simulink model "Sine_Cases"  (R2023a)
settings: Solver=VariableStepAuto  StartTime=0.0  StopTime=10  RelTol=1e-3
settings Model: Creator=HP  LastModifiedBy=HP

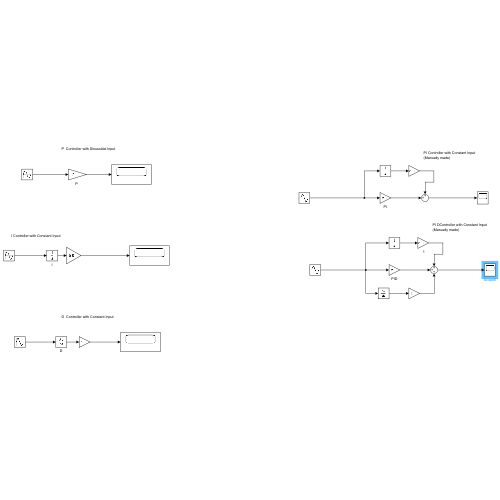
[thumbnail: Simulink's stored preview of the top-level diagram]
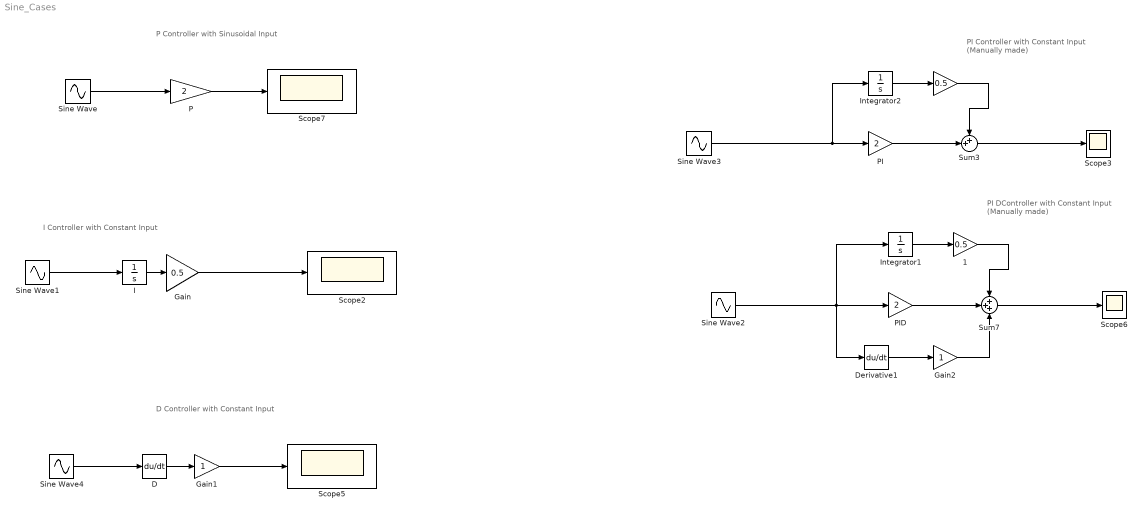
== system Sine_Cases ==
  note: D Controller with Constant Input
  note: PI Controller with Constant Input
      | (Manually made)
  note: I Controller with Constant Input
  note: P Controller with Sinusoidal Input
  note: PI DController with Constant Input
      | (Manually made)
  " " : Gain  Gain=0.5
  " 1" : Gain  Gain=0.5
  D : Derivative
  Derivative1 : Derivative
  Gain : Gain  Gain=0.5
  Gain1 : Gain
  Gain2 : Gain
  I : Integrator
  Integrator1 : Integrator
  Integrator2 : Integrator
  "P  " : Gain  Gain=2
  PI : Gain  Gain=2
  PID : Gain  Gain=2
  Scope{2..3,5..7} (5 alike) : Scope
  Sine Wave{,1..4} (5 alike) : Sin  Amplitude=5  SampleTime=0
  Sum3 : Sum  Inputs=++|
  Sum7 : Sum  Inputs=+++
  wires:
  Gain1/1 -> Scope5/1
  Integrator1/1 -> " 1"/1
  "P  "/1 -> Scope7/1
  Gain/1 -> Scope2/1
  Sine Wave3/1 -> Integrator2/1, PI/1
  Derivative1/1 -> Gain2/1
  Gain2/1 -> Sum7/3
  Sine Wave4/1 -> D/1
  I/1 -> Gain/1
  Sine Wave/1 -> "P  "/1
  D/1 -> Gain1/1
  Integrator2/1 -> " "/1
  Sum3/1 -> Scope3/1
  Sine Wave1/1 -> I/1
  Sine Wave2/1 -> Derivative1/1, PID/1, Integrator1/1
  Sum7/1 -> Scope6/1
  " 1"/1 -> Sum7/1
  PID/1 -> Sum7/2
  PI/1 -> Sum3/2
  " "/1 -> Sum3/1
